simulink model "BE_simu3"  (R2022b)
settings: Solver=VariableStepAuto  StartTime=0.0  StopTime=10  RelTol=1e-3
values from neighbouring files (symbols this model uses):
  Np = 52    [BE_eletr.m]
settings Model: Creator=antoi  LastModifiedBy=guilhermepifferchristo
settings SolverCC: AlgebraicLoopSolver=TrustRegion
settings DebuggingCC: UnconnectedInputMsg=warning  UnconnectedOutputMsg=warning  UnconnectedLineMsg=warning  SFMachineParentedDataDiag=warning  ArithmeticOperatorsInVariantConditions=warning
settings ModelReferenceCC: EnableRefExpFcnMdlSchedulingChecks=on
settings SFSimCC: CustomCodeUndefinedFunction=UseInterfaceOnly

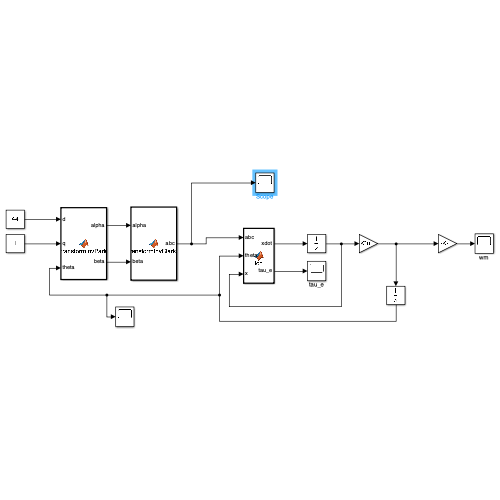
[thumbnail: Simulink's stored preview of the top-level diagram]
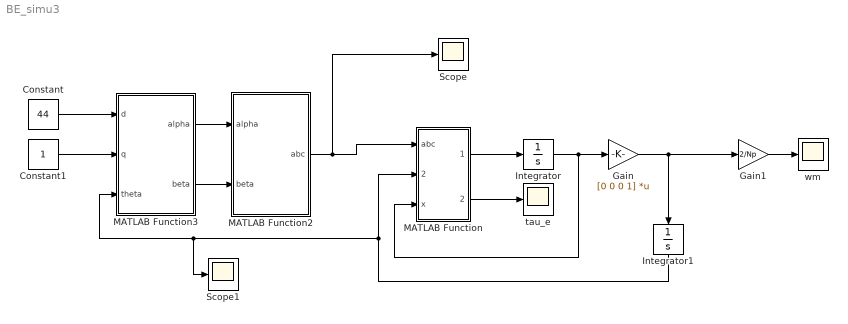
== system BE_simu3 ==
  Constant : Constant  Value=44
  Constant1 : Constant
  Gain : Gain  Gain=[0 0 0 1]  Multiplication=Matrix(K*u)
  Gain1 : Gain  Gain=2/Np
  Integrator : Integrator  InitialCondition=[0 ;0 ;0;0]
  Integrator1 : Integrator
  MATLAB Function : MATLAB Function  TreatAsAtomicUnit=on
  MATLAB Function2 : MATLAB Function  TreatAsAtomicUnit=on
  MATLAB Function3 : MATLAB Function  TreatAsAtomicUnit=on
  Scope : Scope
  Scope1 : Scope
  tau_e : Scope
  wm : Scope
  wires:
  MATLAB Function/2(tau_e) -> tau_e/1
  Integrator/1 -> MATLAB Function/3(x), Gain/1
  MATLAB Function/1(xdot) -> Integrator/1
  Gain1/1 -> wm/1
  Gain/1 -> Integrator1/1, Gain1/1
  Integrator1/1 -> Scope1/1, MATLAB Function3/3(theta), MATLAB Function/2(theta)
  MATLAB Function3/2(beta) -> MATLAB Function2/2(beta)
  MATLAB Function3/1(alpha) -> MATLAB Function2/1(alpha)
  MATLAB Function2/1(abc) -> Scope/1, MATLAB Function/1(abc)
  Constant/1 -> MATLAB Function3/1(d)
  Constant1/1 -> MATLAB Function3/2(q)

== matlab function BE_simu3/MATLAB Function ==
  data: abc input; xdot output; theta input; x input; tau_e output
function [xdot,tau_e] = fcn(abc,theta,x)
    va = abc(1);
    vb = abc(2);
    vc = abc(3);

    Rs = 0.124 ;
    Ls = 0.0021 ;
    lambm = 0.0744 ;
    Np = 52 ;
    M = 92 ;
    Rw = 0.33 ;
    Jt = M*Rw*Rw ;
    Ca = 0.18 ;
    s = 0.05 ;
    tau_c = 0 ;
    g = 9.81 ;

    tau_e = (Np/2)*(x(1)*lambm*(-sin(theta))+x(2)*lambm*(-sin(theta-2*pi/3))+x(3)*lambm*(-sin(theta+2*pi/3)));
    tau_load = (M*g*s*Rw + Ca*Rw*Rw*Rw*x(4)*x(4)*4/(Np*Np)) ;

    xdot1 = va/Ls - (Rs/Ls)*x(1) + (lambm/Ls)*x(4)*sin(theta) ; 
    xdot2 = vb/Ls - (Rs/Ls)*x(2) + (lambm/Ls)*x(4)*sin(theta -2*pi/3) ;
    xdot3 = vc/Ls - (Rs/Ls)*x(3) + (lambm/Ls)*x(4)*sin(theta +2*pi/3) ;
    xdot4 = (Np/(2*Jt))*(tau_e - tau_load + tau_c)  ;
    xdot=[xdot1;xdot2;xdot3;xdot4] ;
end

== matlab function BE_simu3/MATLAB Function2 ==
  data: alpha input; abc output; beta input
function abc  = transformInvClarke(alpha, beta)
    T_clarke_inv = sqrt(2/3) * [1, 0; -1/2, sqrt(3)/2; -1/2, -sqrt(3)/2];
    
    alpha_beta = [alpha; beta];
    abc = T_clarke_inv * alpha_beta;
end

== matlab function BE_simu3/MATLAB Function3 ==
  data: d input; alpha output; q input; theta input; beta output
function [alpha, beta] = transformInvPark(d, q, theta)
    T_park_inv = inv([cos(theta) sin(theta); -sin(theta) cos(theta)]);
    
    dq = [d; q];
    alpha_beta = T_park_inv * dq;
    
    alpha = alpha_beta(1);
    beta = alpha_beta(2);
end
